simulink model "etc_demo_simlink"  (R2017a)
settings: Solver=VariableStepAuto  StartTime=0.0  StopTime=1  RelTol=1e-3
values from neighbouring files (symbols this model uses):
  B = 0.0088    [sim_demo_set_para.m]
  J = 0.0021    [sim_demo_set_para.m]
  K = 0.383    [sim_demo_set_para.m]
  Ks = 0.087    [sim_demo_set_para.m]
  L = 1.5e-3    (= 0.0015)    [sim_demo_set_para.m]
  R = 1.5    [sim_demo_set_para.m]
  Tf = 0    [sim_demo_set_para.m]
  Tpl = 0.396    [sim_demo_set_para.m]
libraries: simulink x1
settings Model: Creator=xiaopan  LastModifiedBy=xiaopan

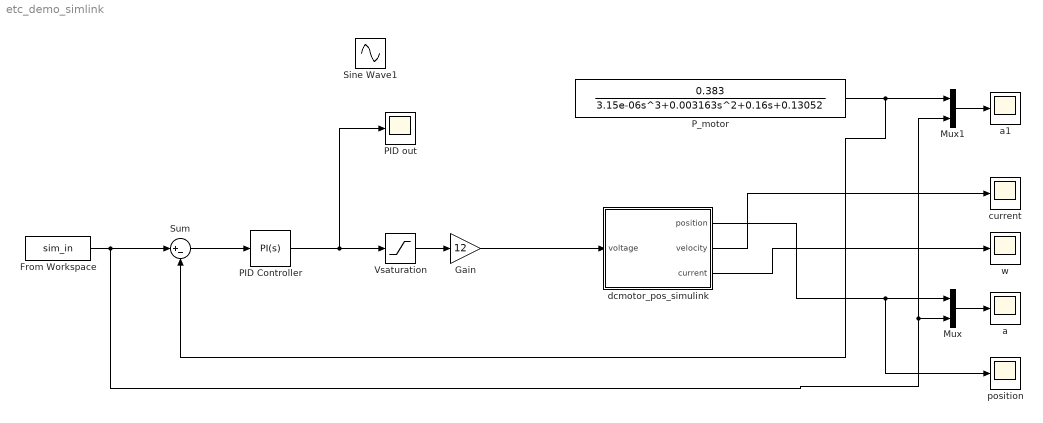
== system etc_demo_simlink ==
  From Workspace : FromWorkspace  VariableName=sim_in  OutDataTypeStr=double  SampleTime=0  OutputAfterFinalValue=Holding final value
  Gain : Gain  Gain=12
  Mux : Mux  Inputs=2
  Mux1 : Mux  Inputs=2
  PID Controller : simulink/Continuous/PID Controller  Controller=PI  TimeDomain=Continuous-time  SampleTime=-1  IntegratorMethod=Forward Euler  FilterMethod=Forward Euler  Form=Parallel  UseFilter=on  ControllerParametersSource=internal  P=5.75  I=16.75  D=0  N=100  InitialConditionSource=internal  InitialConditionForIntegrator=0  InitialConditionForFilter=0  ExternalReset=none  LimitOutput=off  UpperSaturationLimit=inf  LowerSaturationLimit=-inf  LinearizeAsGain=on  AntiWindupMode=none  Kb=1  TrackingMode=off  Kt=1  PParamMin=[]  PParamMax=[]  IParamMin=[]  IParamMax=[]  DParamMin=[]  DParamMax=[]  NParamMin=[]  NParamMax=[]  KbParamMin=[]  KbParamMax=[]  KtParamMin=[]  KtParamMax=[]  POutMin=[]  POutMax=[]  IOutMin=[]  IOutMax=[]  DOutMin=[]  DOutMax=[]  NOutMin=[]  NOutMax=[]  KbOutMin=[]  KbOutMax=[]  KtOutMin=[]  KtOutMax=[]  IntegratorOutMin=[]  IntegratorOutMax=[]  FilterOutMin=[]  FilterOutMax=[]  SumOutMin=[]  SumOutMax=[]  SumI1OutMin=[]  SumI1OutMax=[]  SumI2OutMin=[]  SumI2OutMax=[]  SumI3OutMin=[]  SumI3OutMax=[]  SumDOutMin=[]  SumDOutMax=[]  SaturationOutMin=[]  SaturationOutMax=[]  IntegratorContinuousStateAttributes=''  IntegratorStateMustResolveToSignalObject=off  IntegratorRTWStateStorageClass=Auto  FilterContinuousStateAttributes=''  FilterStateMustResolveToSignalObject=off  FilterRTWStateStorageClass=Auto  DifferentiatorICPrevScaledInput=0  DifferentiatorOutMin=[]  DifferentiatorOutMax=[]  InitialConditionSetting=State (most efficient)
  PID out : Scope
  P_motor : TransferFcn  Numerator=[0.383]  Denominator="[ 3.15e-06  0.003163  0.16  0.13052]"
  Sine Wave1 : Sin  Amplitude=5  Bias=5  Frequency=62.8  SampleTime=0
  Sum : Sum  Inputs=|+-
  Vsaturation : Saturate  UpperLimit=1  LowerLimit=0
  a : Scope
  a1 : Scope
  current : Scope
  dcmotor_pos_simulink : Subsystem
  position : Scope
  w : Scope
  wires:
  Mux/1 -> a/1
  Mux1/1 -> a1/1
  Vsaturation/1 -> Gain/1
  PID Controller/1 -> Vsaturation/1, PID out/1
  P_motor/1 -> Sum/2, Mux1/1
  Sum/1 -> PID Controller/1
  dcmotor_pos_simulink/2(velocity) -> current/1
  dcmotor_pos_simulink/3(current) -> w/1
  From Workspace/1 -> Mux1/2, Mux/2, Sum/1
  dcmotor_pos_simulink/1(position) -> position/1, Mux/1
  Gain/1 -> dcmotor_pos_simulink/1(voltage)

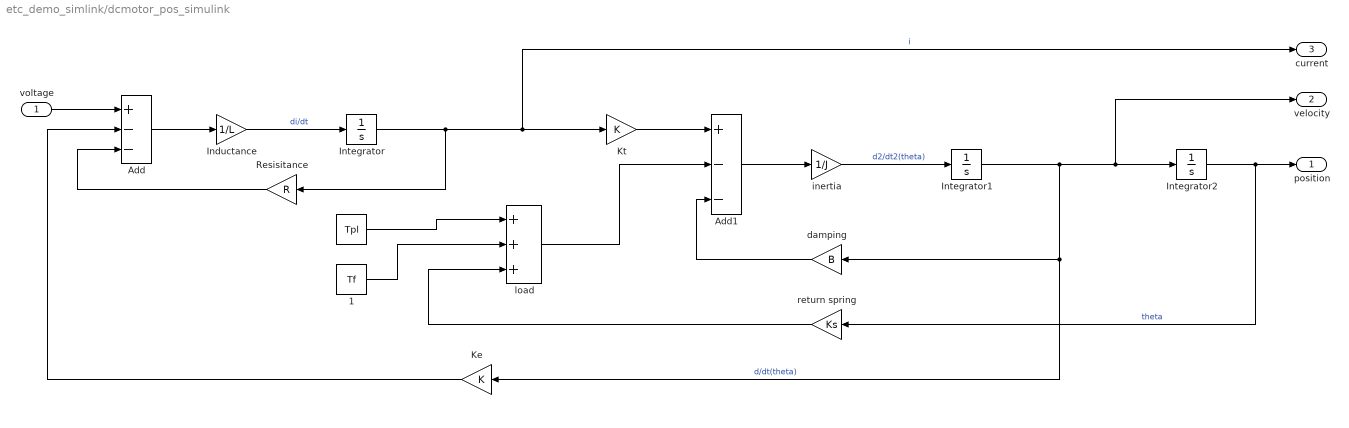
== system etc_demo_simlink/dcmotor_pos_simulink ==
  voltage : Inport
  " " : Constant  Value=Tpl
  " 1" : Constant  Value=Tf
  Add : Sum  Inputs=+--
  Add1 : Sum  Inputs=+--
  "Inductance " : Gain  Gain=1/L
  Integrator : Integrator
  Integrator1 : Integrator
  Integrator2 : Integrator
  Ke : Gain  Gain=K
  Kt : Gain  Gain=K
  Resisitance : Gain  Gain=R
  damping : Gain  Gain=B
  inertia : Gain  Gain=1/J
  load : Sum  Inputs=+++
  return spring : Gain  Gain=Ks
  position : Outport
  velocity : Outport  Port=2
  current : Outport  Port=3
  wires:
  Kt/1 -> Add1/1
  Add/1 -> "Inductance "/1
  "Inductance "/1 -> Integrator/1  "di/dt"
  Integrator2/1 -> position/1, return spring/1  "theta"
  inertia/1 -> Integrator1/1  "d2/dt2(theta)"
  Integrator1/1 -> Integrator2/1, velocity/1, Ke/1, damping/1  "d/dt(theta)"
  Integrator/1 -> Resisitance/1, current/1, Kt/1  "i"
  Add1/1 -> inertia/1
  " "/1 -> load/1
  " 1"/1 -> load/2
  return spring/1 -> load/3
  damping/1 -> Add1/3
  load/1 -> Add1/2
  Ke/1 -> Add/2
  voltage/1 -> Add/1
  Resisitance/1 -> Add/3
